simulink model "detumbling"  (R2020b)
settings: Solver=ode15s  StartTime=0  StopTime=10000  MaxStep=0.1  RelTol=1e-8  AbsTol=1e-8
values from neighbouring files (symbols this model uses):
  data = struct()    [config.m]    (also in config6U.m; configSlew.m; mainOffNominal.m = dataFix)
libraries: simulink_extras x1
settings Model: SimulationMode=accelerator  Creator=pacif  LastModifiedBy=pacif

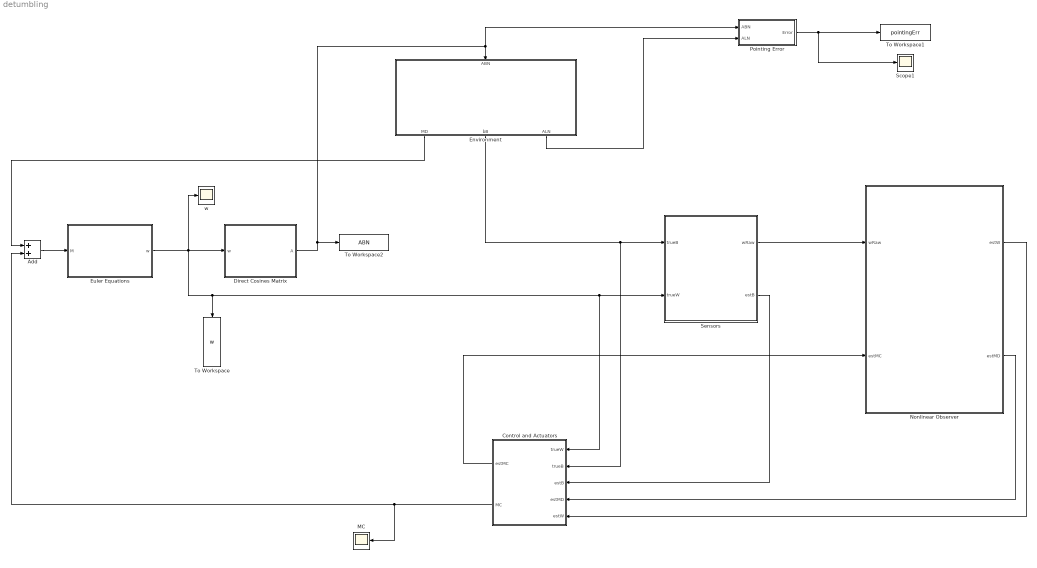
== system detumbling ==
  Add : Sum
  Control and Actuators : Subsystem
  Direct Cosines Matrix : Subsystem
  Environment : Subsystem
  Euler Equations : Subsystem
  MC : Scope
  Nonlinear Observer : Subsystem
  Pointing Error : Subsystem
  Scope1 : Scope
  Sensors : Subsystem
  To Workspace : ToWorkspace  VariableName=w  SaveFormat=Timeseries  SampleTime=-1
  To Workspace1 : ToWorkspace  VariableName=pointingErr  SaveFormat=Timeseries  SampleTime=-1
  To Workspace2 : ToWorkspace  VariableName=ABN  SaveFormat=Timeseries  SampleTime=-1
  w : Scope
  wires:
  Environment/2(bB) -> Sensors/1(trueB), Control and Actuators/2(trueB)
  Add/1 -> Euler Equations/1(M)
  Environment/1(MD) -> Add/1
  Control and Actuators/2(MC) -> MC/1, Add/2
  Sensors/2(estB) -> Control and Actuators/3(estB)
  Sensors/1(wRaw) -> Nonlinear Observer/1(wRaw)
  Control and Actuators/1(estMC) -> Nonlinear Observer/2(estMC)
  Nonlinear Observer/2(estMD) -> Control and Actuators/4(estMD)
  Euler Equations/1(w) -> w/1, Direct Cosines Matrix/1(w), To Workspace/1, Control and Actuators/1(trueW), Sensors/2(trueW)
  Nonlinear Observer/1(estW) -> Control and Actuators/5(estW)
  Pointing Error/1(Error) -> Scope1/1, To Workspace1/1
  Environment/3(ALN) -> Pointing Error/2(ALN)
  Direct Cosines Matrix/1(A) -> Pointing Error/1(ABN), Environment/1(ABN), To Workspace2/1

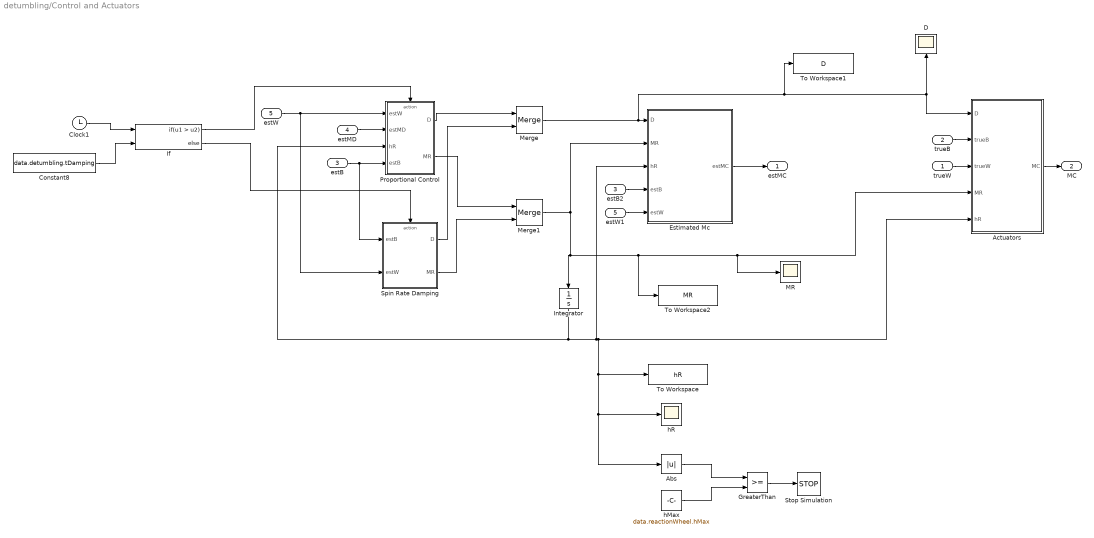
== system detumbling/Control and Actuators ==
  trueW : Inport
  trueB : Inport  Port=2
  estB : Inport  Port=3
  estMD : Inport  Port=4
  estW : Inport  Port=5
  Abs : Abs
  Actuators : Subsystem
  Clock1 : Clock
  Constant8 : Constant  Value=data.detumbling.tDamping
  D : Scope
  Estimated Mc : Subsystem
  GreaterThan : RelationalOperator  OutDataTypeStr=boolean  RndMeth=Simplest
  If : If  NumInputs=2  IfExpression=u1 > u2
  Integrator : Integrator  InitialCondition=data.reactionWheel.h0
  MR : Scope
  Merge : Merge
  Merge1 : Merge
  Proportional Control : Subsystem  TreatAsAtomicUnit=on
  Spin Rate Damping : Subsystem  TreatAsAtomicUnit=on
  Stop Simulation : Stop
  To Workspace : ToWorkspace  VariableName=hR  SaveFormat=Timeseries  SampleTime=-1
  To Workspace1 : ToWorkspace  VariableName=D  SaveFormat=Timeseries  SampleTime=-1
  To Workspace2 : ToWorkspace  VariableName=MR  SaveFormat=Timeseries  SampleTime=-1
  estB2 : InportShadow  Port=3
  estW1 : InportShadow  Port=5
  hMax : Constant  Value=data.reactionWheel.hMax
  hR : Scope
  estMC : Outport
  MC : Outport  Port=2
  wires:
  trueB/1 -> Actuators/2(trueB)
  Actuators/1(MC) -> MC/1
  trueW/1 -> Actuators/3(trueW)
  Merge/1 -> To Workspace1/1, Actuators/1(D), D/1, Estimated Mc/1(D)
  Estimated Mc/1(estMC) -> estMC/1
  Merge1/1 -> To Workspace2/1, Actuators/4(MR), MR/1, Integrator/1, Estimated Mc/2(MR)
  Spin Rate Damping/1(D) -> Merge/2
  Constant8/1 -> If/2
  If/2 -> Spin Rate Damping/Action
  Proportional Control/2(MR) -> Merge1/1
  estB/1 -> Spin Rate Damping/1(estB), Proportional Control/4(estB)
  estW/1 -> Proportional Control/1(estW), Spin Rate Damping/2(estW)
  Clock1/1 -> If/1
  If/1 -> Proportional Control/Action
  estMD/1 -> Proportional Control/2(estMD)
  Proportional Control/1(D) -> Merge/1
  Spin Rate Damping/2(MR) -> Merge1/2
  estB2/1 -> Estimated Mc/4(estB)
  estW1/1 -> Estimated Mc/5(estW)
  Abs/1 -> GreaterThan/1
  GreaterThan/1 -> Stop Simulation/1
  hMax/1 -> GreaterThan/2
  Integrator/1 -> Actuators/5(hR), To Workspace/1, Abs/1, hR/1, Estimated Mc/3(hR), Proportional Control/3(hR)

== system detumbling/Direct Cosines Matrix ==
  w : Inport
  Build 3x3 Matrix : Subsystem
  Constant1 : Constant  Value=0
  Demux1 : Demux  Outputs=3
  Gain{3,5..7} (4 alike) : Gain  Gain=-1
  Integrator : Integrator  InitialCondition=data.ic.dcm
  Orthonormalization : Subsystem
  Product : Product  Multiplication=Matrix(*)
  A : Outport
  wires:
  Demux1/1 -> Build 3x3 Matrix/6(A32), Gain7/1
  Gain5/1 -> Build 3x3 Matrix/4(A12)
  Demux1/3 -> Build 3x3 Matrix/2(A21), Gain5/1
  Product/1 -> Gain3/1
  Build 3x3 Matrix/1(A) -> Product/1  "[w]^"
  Gain6/1 -> Build 3x3 Matrix/3(A31)
  Demux1/2 -> Build 3x3 Matrix/7("A13 "), Gain6/1
  Gain7/1 -> Build 3x3 Matrix/8(A23)
  Orthonormalization/1(A) -> Product/2, A/1
  Gain3/1 -> Integrator/1  "dA/dt"
  w/1 -> Demux1/1
  Integrator/1 -> Orthonormalization/1(A0)  "A"
  Constant1/1 -> Build 3x3 Matrix/1(A11), Build 3x3 Matrix/9(A33), Build 3x3 Matrix/5(A22)

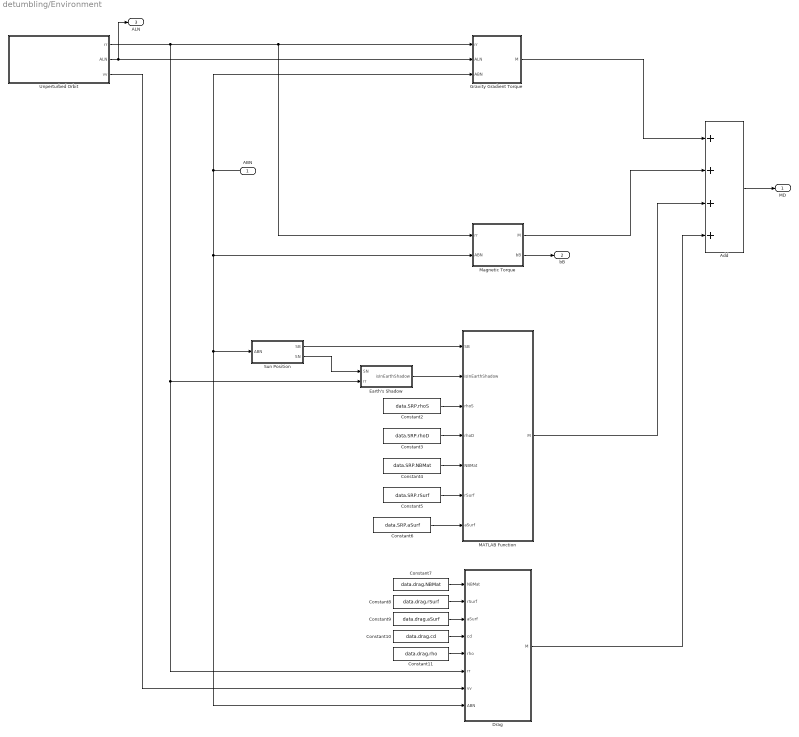
== system detumbling/Environment ==
  ABN : Inport
  Add : Sum  Inputs=++++
  Constant10 : Constant  Value=data.drag.cd
  Constant11 : Constant  Value=data.drag.rho
  Constant2 : Constant  Value=data.SRP.rhoS
  Constant3 : Constant  Value=data.SRP.rhoD
  Constant4 : Constant  Value=data.SRP.NBMat
  Constant5 : Constant  Value=data.SRP.rSurf
  Constant6 : Constant  Value=data.SRP.aSurf
  Constant7 : Constant  Value=data.drag.NBMat
  Constant8 : Constant  Value=data.drag.rSurf
  Constant9 : Constant  Value=data.drag.aSurf
  Drag : MATLAB Function  TreatAsAtomicUnit=on
  Earth's Shadow : Subsystem
  Gravity Gradient Torque : Subsystem
  MATLAB Function : MATLAB Function  TreatAsAtomicUnit=on
  Magnetic Torque : Subsystem
  "Sun Position " : Subsystem
  Unperturbed Orbit : Subsystem
  MD : Outport
  bB : Outport  Port=2
  ALN : Outport  Port=3
  wires:
  Earth's Shadow/1(isInEarthShadow) -> MATLAB Function/2(isInEarthShadow)
  "Sun Position "/1(SB) -> MATLAB Function/1(SB)
  Constant5/1 -> MATLAB Function/6(rSurf)
  Constant6/1 -> MATLAB Function/7(aSurf)
  Constant3/1 -> MATLAB Function/4(rhoD)
  Constant4/1 -> MATLAB Function/5(NBMat)
  Gravity Gradient Torque/1(M) -> Add/1
  Unperturbed Orbit/1(rr) -> Earth's Shadow/2(rr), Drag/6(rr), Magnetic Torque/1(rr), Gravity Gradient Torque/1(rr)
  MATLAB Function/1(M) -> Add/3
  Constant10/1 -> Drag/4(cd)
  Drag/1(M) -> Add/4
  ABN/1 -> Gravity Gradient Torque/3(ABN), Magnetic Torque/2(ABN), Drag/8(ABN), "Sun Position "/1(ABN)
  Constant7/1 -> Drag/1(NBMat)
  Constant8/1 -> Drag/2(rSurf)
  Constant9/1 -> Drag/3(aSurf)
  Add/1 -> MD/1
  Constant2/1 -> MATLAB Function/3(rhoS)
  Magnetic Torque/1(M) -> Add/2
  Unperturbed Orbit/2(ALN) -> Gravity Gradient Torque/2(ALN), ALN/1
  Constant11/1 -> Drag/5(rho)
  Unperturbed Orbit/3(vv) -> Drag/7(vv)
  Magnetic Torque/2(bB) -> bB/1
  "Sun Position "/2(SN) -> Earth's Shadow/1(SN)

== system detumbling/Euler Equations ==
  M : Inport
  Add : Sum
  Cross Product : Subsystem
  Gain : Gain  Gain=data.sc.invI  Multiplication=Matrix(K*u) (u vector)
  Gain2 : Gain  Gain=data.sc.inertiaMatrix  Multiplication=Matrix(K*u) (u vector)
  Integrator : Integrator  InitialCondition=data.ic.w
  w : Outport
  wires:
  Gain2/1 -> Cross Product/1(a)  "I*w"
  Cross Product/1(c) -> Add/2  "I*w x w = -w x I*w"
  M/1 -> Add/1
  Integrator/1 -> Cross Product/2(b), Gain2/1, w/1  "w"
  Gain/1 -> Integrator/1  "dw"
  Add/1 -> Gain/1

== system detumbling/Nonlinear Observer ==
  wRaw : Inport
  estMC : Inport  Port=2
  Observer : Subsystem
  estW : Outport
  estMD : Outport  Port=2
  wires:
  wRaw/1 -> Observer/1(wRaw)
  estMC/1 -> Observer/2(estMC)
  Observer/1(estW) -> estW/1
  Observer/2(estMD) -> estMD/1

== system detumbling/Pointing Error ==
  ABN : Inport
  ALN : Inport  Port=2
  Acos : Trigonometry  Operator=acos
  Product : Product  Multiplication=Matrix(*)
  Radians to Degrees : simulink_extras/Transformations/Radians to Degrees
  Selector : Selector  NumberOfDimensions=2  InputPortWidth=3  IndexOptions=Index vector (dialog),Index vector (dialog)  Indices=1,1  OutputSizes=1,1
  Transpose : Math  Operator=transpose  SaturateOnIntegerOverflow=on
  Error : Outport
  wires:
  Radians to Degrees/1 -> Error/1
  ABN/1 -> Product/1
  ALN/1 -> Transpose/1
  Transpose/1 -> Product/2
  Product/1 -> Selector/1
  Selector/1 -> Acos/1
  Acos/1 -> Radians to Degrees/1

== system detumbling/Sensors ==
  trueB : Inport
  trueW : Inport  Port=2
  Add3 : Sum  Inputs=+-
  Gyro Error : Scope
  Gyroscope : Subsystem
  Magnetometer : Subsystem
  wRaw : Outport
  estB : Outport  Port=2
  wires:
  Gyroscope/1(wRaw) -> wRaw/1, Add3/2
  trueW/1 -> Add3/1, Gyroscope/1(trueW)
  Add3/1 -> Gyro Error/1
  Magnetometer/1(estB) -> estB/1
  trueB/1 -> Magnetometer/1(B)

== system detumbling/Control and Actuators/Actuators ==
  D : Inport
  trueB : Inport  Port=2
  trueW : Inport  Port=3
  MR : Inport  Port=4
  hR : Inport  Port=5
  Add : Sum
  Add1 : Sum
  Cross Product : Subsystem
  Cross Product1 : Subsystem
  Gain : Gain  Gain=-1
  Product : Product
  Product1 : Product
  Reaction Wheel Axis : Constant  Value=data.reactionWheel.axis
  MC : Outport
  wires:
  D/1 -> Cross Product/1(a)
  trueB/1 -> Cross Product/2(b)
  Add/1 -> MC/1
  Cross Product/1(c) -> Add/1
  Gain/1 -> Add/2
  Add1/1 -> Gain/1
  Cross Product1/1(c) -> Add1/1
  trueW/1 -> Cross Product1/1(a)
  Product/1 -> Cross Product1/2(b)
  MR/1 -> Product1/2
  hR/1 -> Product/1
  Reaction Wheel Axis/1 -> Product1/1, Product/2
  Product1/1 -> Add1/2

== system detumbling/Control and Actuators/Estimated Mc ==
  D : Inport
  MR : Inport  Port=2
  hR : Inport  Port=3
  estB : Inport  Port=4
  estW : Inport  Port=5
  Add : Sum  Inputs=+--
  Cross Product : Subsystem
  Cross Product1 : Subsystem
  Product : Product
  Product1 : Product
  RW Axis : Constant  Value=data.reactionWheel.axis
  RW Axis1 : Constant  Value=data.reactionWheel.axis
  estMC : Outport
  wires:
  D/1 -> Cross Product/1(a)
  estB/1 -> Cross Product/2(b)
  Add/1 -> estMC/1
  Cross Product/1(c) -> Add/1
  RW Axis/1 -> Product/1
  MR/1 -> Product/2
  Product/1 -> Add/2
  Cross Product1/1(c) -> Add/3
  estW/1 -> Cross Product1/1(a)
  hR/1 -> Product1/2
  RW Axis1/1 -> Product1/1
  Product1/1 -> Cross Product1/2(b)

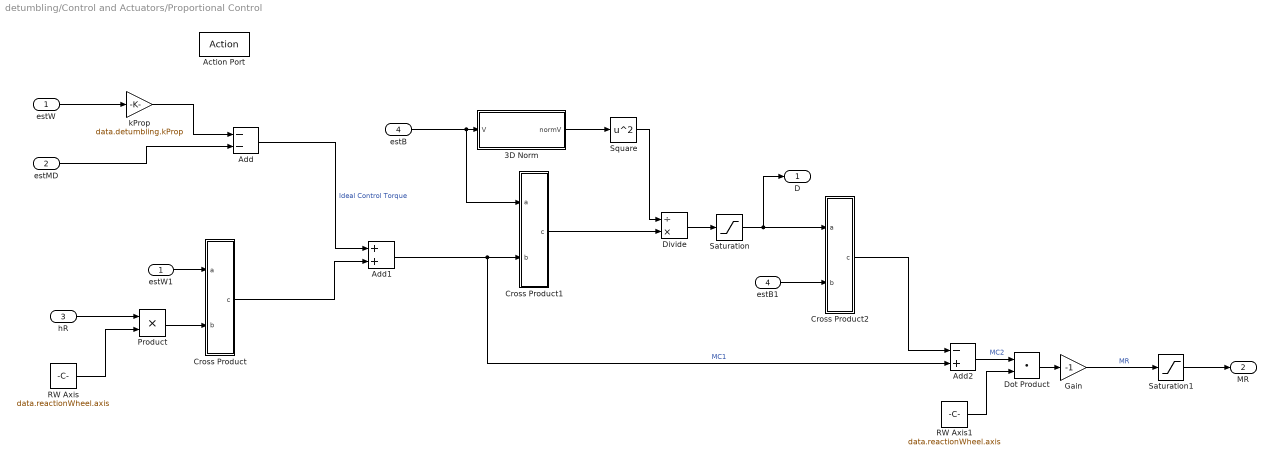
== system detumbling/Control and Actuators/Proportional Control ==
  estW : Inport
  estMD : Inport  Port=2
  hR : Inport  Port=3
  estB : Inport  Port=4
  Action Port : ActionPort  ActionPortLabel=if(u1 > u2)
  3D Norm : Subsystem
  Add : Sum  Inputs=--
  Add1 : Sum
  Add2 : Sum  Inputs=-+
  Cross Product : Subsystem
  Cross Product1 : Subsystem
  Cross Product2 : Subsystem
  Divide : Product  Inputs=/*
  Dot Product : DotProduct  InputSameDT=on  OutDataTypeStr=Inherit: Inherit via internal rule
  Gain : Gain  Gain=-1
  Product : Product
  RW Axis : Constant  Value=data.reactionWheel.axis
  RW Axis1 : Constant  Value=data.reactionWheel.axis
  Saturation : Saturate  UpperLimit=data.magnetorquer.DMax  LowerLimit=-data.magnetorquer.DMax  LinearizeAsGain=off
  Saturation1 : Saturate  UpperLimit=data.reactionWheel.MMax  LowerLimit=-data.reactionWheel.MMax
  Square : Math  Operator=square  SaturateOnIntegerOverflow=on
  estB1 : InportShadow  Port=4
  estW1 : InportShadow
  kProp : Gain  Gain=data.detumbling.kProp
  D : Outport
  MR : Outport  Port=2
  wires:
  Saturation/1 -> Cross Product2/1(a), D/1
  Divide/1 -> Saturation/1
  estW/1 -> kProp/1
  kProp/1 -> Add/1
  estMD/1 -> Add/2
  Add/1 -> Add1/1  "Ideal Control Torque"
  estW1/1 -> Cross Product/1(a)
  Product/1 -> Cross Product/2(b)
  hR/1 -> Product/1
  RW Axis/1 -> Product/2
  Cross Product/1(c) -> Add1/2
  estB/1 -> Cross Product1/1(a), 3D Norm/1(V)
  3D Norm/1(normV) -> Square/1
  Add1/1 -> Cross Product1/2(b), Add2/2  "MC1"
  Cross Product1/1(c) -> Divide/2
  Square/1 -> Divide/1
  estB1/1 -> Cross Product2/2(b)
  Cross Product2/1(c) -> Add2/1
  Add2/1 -> Dot Product/1  "MC2"
  Dot Product/1 -> Gain/1
  RW Axis1/1 -> Dot Product/2
  Gain/1 -> Saturation1/1  "MR"
  Saturation1/1 -> MR/1

== system detumbling/Control and Actuators/Spin Rate Damping ==
  estB : Inport
  estW : Inport  Port=2
  Action Port : ActionPort  ActionPortLabel=else
  Constant : Constant  Value=0
  Cross Product1 : Subsystem
  Saturation : Saturate  UpperLimit=data.magnetorquer.DMax  LowerLimit=-data.magnetorquer.DMax  LinearizeAsGain=off
  k : Gain  Gain=data.detumbling.kDamping
  D : Outport
  MR : Outport  Port=2
  wires:
  estW/1 -> Cross Product1/1(a)
  estB/1 -> Cross Product1/2(b)
  Cross Product1/1(c) -> k/1
  k/1 -> Saturation/1
  Constant/1 -> MR/1
  Saturation/1 -> D/1

== system detumbling/Direct Cosines Matrix/Build 3x3 Matrix ==
  A11 : Inport
  A21 : Inport  Port=2
  A31 : Inport  Port=3
  A12 : Inport  Port=4
  A22 : Inport  Port=5
  A32 : Inport  Port=6
  "A13 " : Inport  Port=7
  A23 : Inport  Port=8
  A33 : Inport  Port=9
  Mux : Mux  Inputs=3
  Mux1 : Mux  Inputs=3
  Mux2 : Mux  Inputs=3
  Vector Concatenate : Concatenate  NumInputs=3  Mode=Multidimensional array  ConcatenateDimension=2
  A : Outport
  wires:
  A21/1 -> Mux/2
  A23/1 -> Mux2/2
  "A13 "/1 -> Mux2/1
  A11/1 -> Mux/1
  Vector Concatenate/1 -> A/1
  A31/1 -> Mux/3
  A12/1 -> Mux1/1
  A22/1 -> Mux1/2
  Mux2/1 -> Vector Concatenate/3
  Mux1/1 -> Vector Concatenate/2
  Mux/1 -> Vector Concatenate/1
  A33/1 -> Mux2/3
  A32/1 -> Mux1/3

== system detumbling/Direct Cosines Matrix/Orthonormalization ==
  A0 : Inport
  Add : Sum  Inputs=+-
  Gain : Gain  Gain=1.5
  Gain1 : Gain  Gain=0.5
  Product : Product  Inputs=3  Multiplication=Matrix(*)
  Transpose : Math  Operator=transpose  SaturateOnIntegerOverflow=on
  A : Outport
  wires:
  Add/1 -> A/1
  A0/1 -> Product/3, Transpose/1, Product/1, Gain/1
  Gain1/1 -> Add/2
  Gain/1 -> Add/1
  Transpose/1 -> Product/2
  Product/1 -> Gain1/1

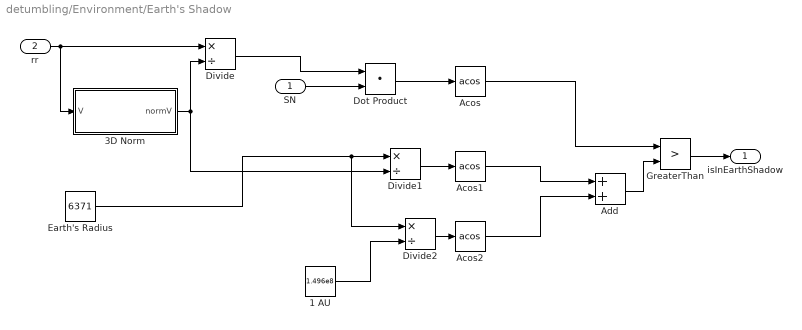
== system detumbling/Environment/Earth's Shadow ==
  SN : Inport
  rr : Inport  Port=2
  1 AU : Constant  Value=1.496e8
  3D Norm : Subsystem
  Acos : Trigonometry  Operator=acos
  Acos1 : Trigonometry  Operator=acos
  Acos2 : Trigonometry  Operator=acos
  Add : Sum
  Divide : Product  Inputs=*/
  Divide1 : Product  Inputs=*/
  Divide2 : Product  Inputs=*/
  Dot Product : DotProduct  InputSameDT=on  OutDataTypeStr=Inherit: Inherit via internal rule
  Earth's Radius : Constant  Value=6371
  GreaterThan : RelationalOperator  Operator=>  OutDataTypeStr=boolean  RndMeth=Simplest
  isInEarthShadow : Outport
  wires:
  SN/1 -> Dot Product/2
  GreaterThan/1 -> isInEarthShadow/1
  Add/1 -> GreaterThan/2
  Acos/1 -> GreaterThan/1
  Acos2/1 -> Add/2
  Acos1/1 -> Add/1
  rr/1 -> 3D Norm/1(V), Divide/1
  3D Norm/1(normV) -> Divide1/2, Divide/2
  Divide/1 -> Dot Product/1
  Dot Product/1 -> Acos/1
  Earth's Radius/1 -> Divide1/1, Divide2/1
  Divide1/1 -> Acos1/1
  Divide2/1 -> Acos2/1
  1 AU/1 -> Divide2/2

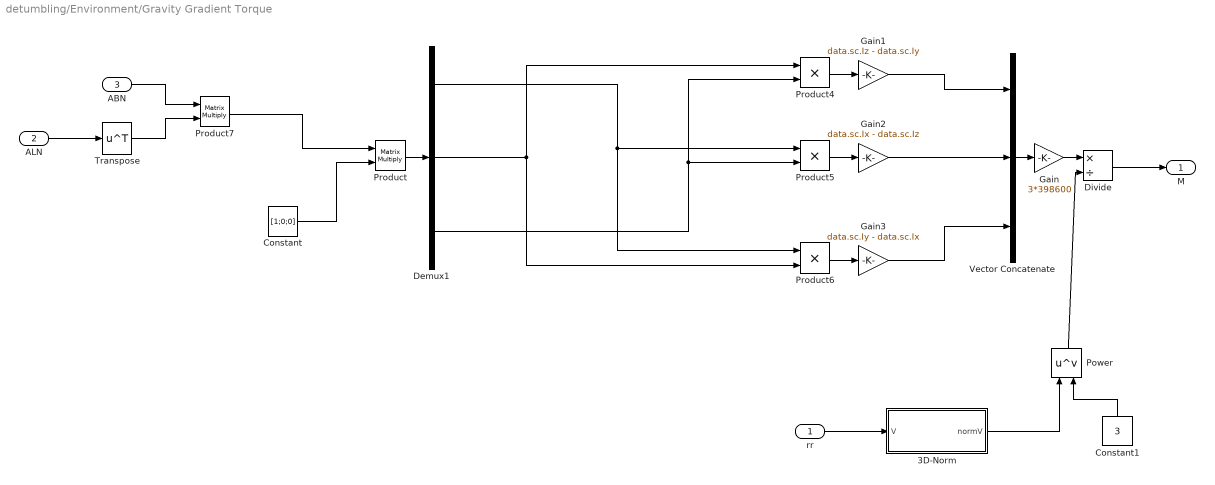
== system detumbling/Environment/Gravity Gradient Torque ==
  rr : Inport
  ALN : Inport  Port=2
  ABN : Inport  Port=3
  3D-Norm : Subsystem
  Constant : Constant  Value=[1;0;0]  VectorParams1D=off
  Constant1 : Constant  Value=3
  Demux1 : Demux  Outputs=3
  Divide : Product  Inputs=*/
  Gain : Gain  Gain=3*398600
  Gain1 : Gain  Gain=data.sc.Iz - data.sc.Iy
  Gain2 : Gain  Gain=data.sc.Ix - data.sc.Iz
  Gain3 : Gain  Gain=data.sc.Iy - data.sc.Ix
  Power : Math  Operator=pow  SaturateOnIntegerOverflow=on
  Product : Product  Multiplication=Matrix(*)
  Product4 : Product
  Product5 : Product
  Product6 : Product
  Product7 : Product  Multiplication=Matrix(*)
  Transpose : Math  Operator=transpose  SaturateOnIntegerOverflow=on
  Vector Concatenate : Concatenate  NumInputs=3
  M : Outport
  wires:
  Constant/1 -> Product/2
  Gain3/1 -> Vector Concatenate/3
  Gain1/1 -> Vector Concatenate/1
  Gain2/1 -> Vector Concatenate/2
  Vector Concatenate/1 -> Gain/1
  Constant1/1 -> Power/2
  Power/1 -> Divide/2
  Gain/1 -> Divide/1
  Product/1 -> Demux1/1
  Product4/1 -> Gain1/1
  Product5/1 -> Gain2/1
  Product6/1 -> Gain3/1
  Demux1/1 -> Product6/1, Product5/1
  Demux1/2 -> Product6/2, Product4/1
  Demux1/3 -> Product5/2, Product4/2
  Divide/1 -> M/1
  rr/1 -> 3D-Norm/1(V)
  3D-Norm/1(normV) -> Power/1
  ALN/1 -> Transpose/1
  Product7/1 -> Product/1
  ABN/1 -> Product7/1
  Transpose/1 -> Product7/2

== system detumbling/Environment/Magnetic Torque ==
  rr : Inport
  ABN : Inport  Port=2
  Cross Product : Subsystem
  Product : Product  Multiplication=Matrix(*)
  Subsystem : Subsystem
  m : Constant  Value=data.magneticTorque.m
  M : Outport
  bB : Outport  Port=2
  wires:
  rr/1 -> Subsystem/1(rr)
  ABN/1 -> Product/1
  Subsystem/1(bN) -> Product/2
  m/1 -> Cross Product/1(a)
  Product/1 -> Cross Product/2(b), bB/1
  Cross Product/1(c) -> M/1

== system detumbling/Environment/Sun Position  ==
  ABN : Inport
  Clock : Clock
  Cos : Trigonometry  Operator=cos
  Gain1 : Gain  Gain=2*pi/365/24/3600
  Gain2 : Gain  Gain=cos(23.45*pi/180)
  Gain3 : Gain  Gain=sin(23.45*pi/180)
  Mux : Mux  Inputs=3
  Product : Product  Multiplication=Matrix(*)
  Sin : Trigonometry
  Sin1 : Trigonometry
  SB : Outport
  SN : Outport  Port=2
  wires:
  Clock/1 -> Gain1/1
  Mux/1 -> SN/1, Product/2  "SN"
  Gain2/1 -> Mux/2
  Gain3/1 -> Mux/3
  Cos/1 -> Mux/1
  Sin1/1 -> Gain3/1
  Sin/1 -> Gain2/1
  Gain1/1 -> Sin/1, Sin1/1, Cos/1
  ABN/1 -> Product/1
  Product/1 -> SB/1

== system detumbling/Environment/Unperturbed Orbit ==
  Integrator : Integrator  InitialCondition=data.ic.th
  Subsystem : Subsystem
  Subsystem1 : Subsystem
  Subsystem2 : Subsystem
  Subsystem3 : Subsystem
  To Workspace : ToWorkspace  VariableName=theta  SaveFormat=Timeseries  SampleTime=-1
  rr : Outport
  ALN : Outport  Port=2
  vv : Outport  Port=3
  wires:
  Subsystem2/1(rr) -> rr/1
  Subsystem/1(theta_dot) -> Integrator/1
  Subsystem1/1(ALN) -> ALN/1
  Subsystem3/1(vv) -> vv/1
  Integrator/1 -> Subsystem2/1(theta), Subsystem1/1(theta), Subsystem3/1(theta), To Workspace/1, Subsystem/1(theta)

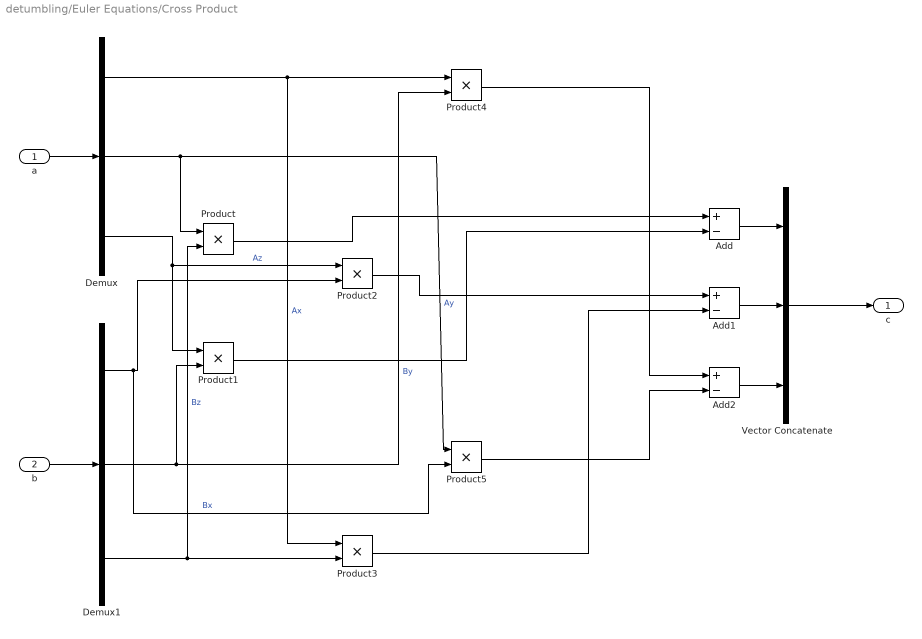
== system detumbling/Euler Equations/Cross Product ==
  a : Inport
  b : Inport  Port=2
  Add : Sum  Inputs=+-
  Add1 : Sum  Inputs=+-
  Add2 : Sum  Inputs=+-
  Demux : Demux  Outputs=3
  Demux1 : Demux  Outputs=3
  Product{,1..5} (6 alike) : Product
  Vector Concatenate : Concatenate  NumInputs=3
  c : Outport
  wires:
  Demux1/1 -> Product2/2, Product5/2  "Bx"
  Product2/1 -> Add1/1
  Vector Concatenate/1 -> c/1
  Add/1 -> Vector Concatenate/1
  Product3/1 -> Add1/2
  Product1/1 -> Add/2
  Product4/1 -> Add2/1
  Product/1 -> Add/1
  Demux/1 -> Product3/1, Product4/1  "Ax"
  Product5/1 -> Add2/2
  Demux/3 -> Product2/1, Product1/1  "Az"
  b/1 -> Demux1/1
  a/1 -> Demux/1
  Add2/1 -> Vector Concatenate/3
  Demux/2 -> Product5/1, Product/1  "Ay"
  Demux1/3 -> Product/2, Product3/2  "Bz"
  Demux1/2 -> Product4/2, Product1/2  "By"
  Add1/1 -> Vector Concatenate/2

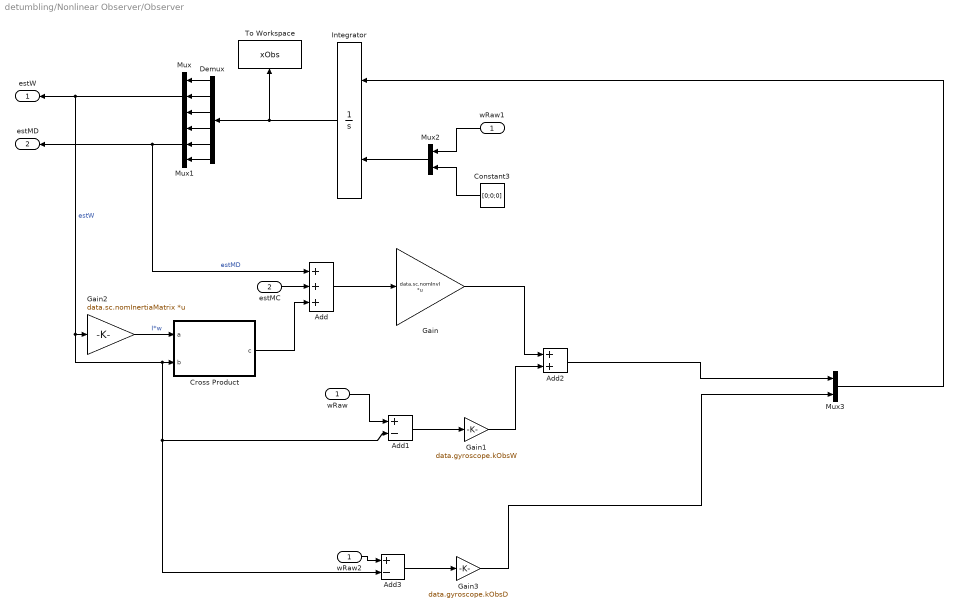
== system detumbling/Nonlinear Observer/Observer ==
  wRaw : Inport
  estMC : Inport  Port=2
  Add : Sum  Inputs=+++
  Add1 : Sum  Inputs=+-
  Add2 : Sum
  Add3 : Sum  Inputs=+-
  Constant3 : Constant  Value=[0;0;0]
  Cross Product : Subsystem
  Demux : Demux  Outputs=6
  Gain : Gain  Gain=data.sc.nomInvI  Multiplication=Matrix(K*u) (u vector)
  Gain1 : Gain  Gain=data.gyroscope.kObsW
  Gain2 : Gain  Gain=data.sc.nomInertiaMatrix  Multiplication=Matrix(K*u) (u vector)
  Gain3 : Gain  Gain=data.gyroscope.kObsD
  Integrator : Integrator  InitialConditionSource=external  InitialCondition=data.gyroscope.xObs0
  Mux : Mux  Inputs=3
  Mux1 : Mux  Inputs=3
  Mux2 : Mux  Inputs=2
  Mux3 : Mux  Inputs=2
  To Workspace : ToWorkspace  VariableName=xObs  SaveFormat=Timeseries  SampleTime=-1
  wRaw1 : InportShadow
  wRaw2 : InportShadow
  estW : Outport
  estMD : Outport  Port=2
  wires:
  Mux3/1 -> Integrator/1
  Integrator/1 -> Demux/1, To Workspace/1
  estMC/1 -> Add/2
  Demux/1 -> Mux/1
  Demux/2 -> Mux/2
  Demux/3 -> Mux/3
  Demux/5 -> Mux1/2
  Demux/4 -> Mux1/1
  Demux/6 -> Mux1/3
  Mux1/1 -> Add/1, estMD/1  "estMD"
  Mux2/1 -> Integrator/2
  wRaw1/1 -> Mux2/1
  Constant3/1 -> Mux2/2
  Cross Product/1(c) -> Add/3
  Add/1 -> Gain/1
  Gain2/1 -> Cross Product/1(a)  "I*w"
  Gain/1 -> Add2/1
  wRaw/1 -> Add1/1
  Add1/1 -> Gain1/1
  Gain1/1 -> Add2/2
  Add2/1 -> Mux3/1
  Add3/1 -> Gain3/1
  Mux/1 -> Add3/2, Add1/2, Cross Product/2(b), Gain2/1, estW/1  "estW"
  Gain3/1 -> Mux3/2
  wRaw2/1 -> Add3/1

== system detumbling/Sensors/Gyroscope ==
  trueW : Inport
  Add : Sum
  Add1 : Sum
  Integrator : Integrator  InitialCondition=data.gyroscope.b0
  Random Number : RandomNumber  Variance=data.gyroscope.sigmaN^2*[1;1;1]  Seed=[2323; 3445;34]  SampleTime=data.gyroscope.sampleTime
  Random Number1 : RandomNumber  Variance=data.gyroscope.sigmaB^2*[1;1;1]  Seed=[34432; 345456;1087]  SampleTime=data.gyroscope.sampleTime
  To Workspace : ToWorkspace  VariableName=bGyro  SaveFormat=Timeseries  SampleTime=-1
  Zero-Order Hold : ZeroOrderHold  SampleTime=data.gyroscope.sampleTime
  wRaw : Outport
  wires:
  Zero-Order Hold/1 -> wRaw/1
  Add/1 -> Zero-Order Hold/1
  Random Number/1 -> Add1/1
  Add1/1 -> Add/2
  trueW/1 -> Add/1
  Integrator/1 -> To Workspace/1, Add1/2
  Random Number1/1 -> Integrator/1

== system detumbling/Sensors/Magnetometer ==
  B : Inport
  Add : Sum
  Multiply : Gain  Gain=data.magnetometer.nonOrthogonality  Multiplication=Matrix(K*u) (u vector)
  Random Number1 : RandomNumber  Variance=(data.magnetometer.sigma)^2*[1;1;1]  Seed=randi(1e5,3,1)  SampleTime=data.magnetometer.sampleTime
  Zero-Order Hold : ZeroOrderHold  SampleTime=data.magnetometer.sampleTime
  estB : Outport
  wires:
  Random Number1/1 -> Add/2
  Add/1 -> Zero-Order Hold/1
  B/1 -> Add/1
  Zero-Order Hold/1 -> Multiply/1
  Multiply/1 -> estB/1

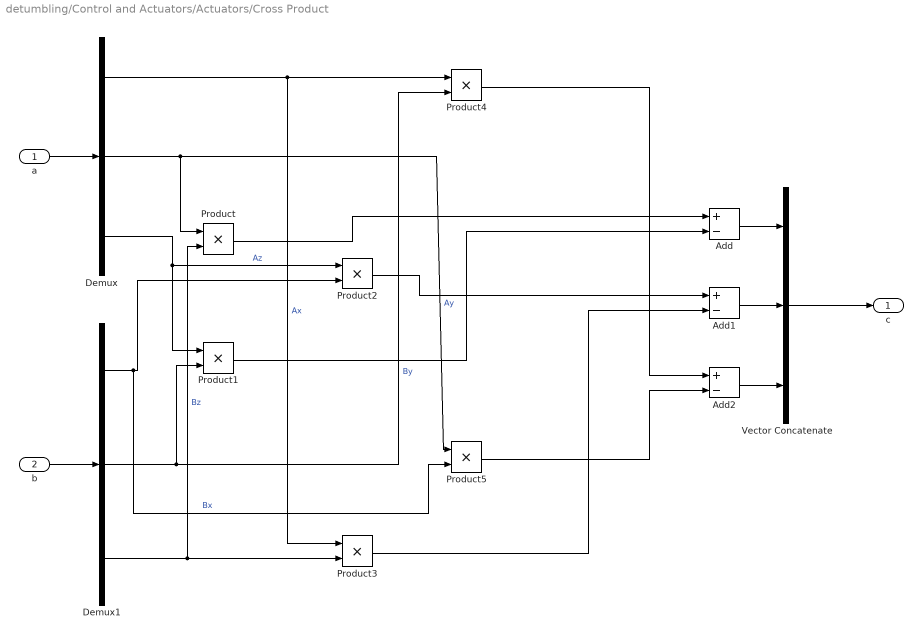
== system detumbling/Control and Actuators/Actuators/Cross Product ==
  a : Inport
  b : Inport  Port=2
  Add : Sum  Inputs=+-
  Add1 : Sum  Inputs=+-
  Add2 : Sum  Inputs=+-
  Demux : Demux  Outputs=3
  Demux1 : Demux  Outputs=3
  Product{,1..5} (6 alike) : Product
  Vector Concatenate : Concatenate  NumInputs=3
  c : Outport
  wires:
  Demux1/1 -> Product2/2, Product5/2  "Bx"
  Product2/1 -> Add1/1
  Vector Concatenate/1 -> c/1
  Add/1 -> Vector Concatenate/1
  Product3/1 -> Add1/2
  Product1/1 -> Add/2
  Product4/1 -> Add2/1
  Product/1 -> Add/1
  Demux/1 -> Product3/1, Product4/1  "Ax"
  Product5/1 -> Add2/2
  Demux/3 -> Product2/1, Product1/1  "Az"
  b/1 -> Demux1/1
  a/1 -> Demux/1
  Add2/1 -> Vector Concatenate/3
  Demux/2 -> Product5/1, Product/1  "Ay"
  Demux1/3 -> Product/2, Product3/2  "Bz"
  Demux1/2 -> Product4/2, Product1/2  "By"
  Add1/1 -> Vector Concatenate/2

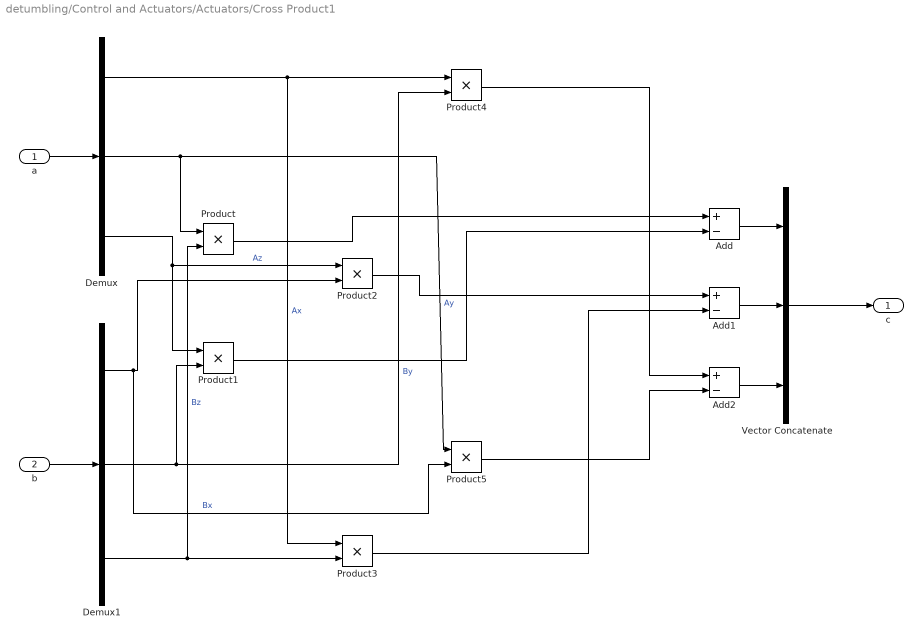
== system detumbling/Control and Actuators/Actuators/Cross Product1 ==
  a : Inport
  b : Inport  Port=2
  Add : Sum  Inputs=+-
  Add1 : Sum  Inputs=+-
  Add2 : Sum  Inputs=+-
  Demux : Demux  Outputs=3
  Demux1 : Demux  Outputs=3
  Product{,1..5} (6 alike) : Product
  Vector Concatenate : Concatenate  NumInputs=3
  c : Outport
  wires:
  Demux1/1 -> Product2/2, Product5/2  "Bx"
  Product2/1 -> Add1/1
  Vector Concatenate/1 -> c/1
  Add/1 -> Vector Concatenate/1
  Product3/1 -> Add1/2
  Product1/1 -> Add/2
  Product4/1 -> Add2/1
  Product/1 -> Add/1
  Demux/1 -> Product3/1, Product4/1  "Ax"
  Product5/1 -> Add2/2
  Demux/3 -> Product2/1, Product1/1  "Az"
  b/1 -> Demux1/1
  a/1 -> Demux/1
  Add2/1 -> Vector Concatenate/3
  Demux/2 -> Product5/1, Product/1  "Ay"
  Demux1/3 -> Product/2, Product3/2  "Bz"
  Demux1/2 -> Product4/2, Product1/2  "By"
  Add1/1 -> Vector Concatenate/2

== system detumbling/Control and Actuators/Estimated Mc/Cross Product ==
  a : Inport
  b : Inport  Port=2
  Add : Sum  Inputs=+-
  Add1 : Sum  Inputs=+-
  Add2 : Sum  Inputs=+-
  Demux : Demux  Outputs=3
  Demux1 : Demux  Outputs=3
  Product{,1..5} (6 alike) : Product
  Vector Concatenate : Concatenate  NumInputs=3
  c : Outport
  wires:
  Demux1/1 -> Product2/2, Product5/2  "Bx"
  Product2/1 -> Add1/1
  Vector Concatenate/1 -> c/1
  Add/1 -> Vector Concatenate/1
  Product3/1 -> Add1/2
  Product1/1 -> Add/2
  Product4/1 -> Add2/1
  Product/1 -> Add/1
  Demux/1 -> Product3/1, Product4/1  "Ax"
  Product5/1 -> Add2/2
  Demux/3 -> Product2/1, Product1/1  "Az"
  b/1 -> Demux1/1
  a/1 -> Demux/1
  Add2/1 -> Vector Concatenate/3
  Demux/2 -> Product5/1, Product/1  "Ay"
  Demux1/3 -> Product/2, Product3/2  "Bz"
  Demux1/2 -> Product4/2, Product1/2  "By"
  Add1/1 -> Vector Concatenate/2

== system detumbling/Control and Actuators/Estimated Mc/Cross Product1 ==
  a : Inport
  b : Inport  Port=2
  Add : Sum  Inputs=+-
  Add1 : Sum  Inputs=+-
  Add2 : Sum  Inputs=+-
  Demux : Demux  Outputs=3
  Demux1 : Demux  Outputs=3
  Product{,1..5} (6 alike) : Product
  Vector Concatenate : Concatenate  NumInputs=3
  c : Outport
  wires:
  Demux1/1 -> Product2/2, Product5/2  "Bx"
  Product2/1 -> Add1/1
  Vector Concatenate/1 -> c/1
  Add/1 -> Vector Concatenate/1
  Product3/1 -> Add1/2
  Product1/1 -> Add/2
  Product4/1 -> Add2/1
  Product/1 -> Add/1
  Demux/1 -> Product3/1, Product4/1  "Ax"
  Product5/1 -> Add2/2
  Demux/3 -> Product2/1, Product1/1  "Az"
  b/1 -> Demux1/1
  a/1 -> Demux/1
  Add2/1 -> Vector Concatenate/3
  Demux/2 -> Product5/1, Product/1  "Ay"
  Demux1/3 -> Product/2, Product3/2  "Bz"
  Demux1/2 -> Product4/2, Product1/2  "By"
  Add1/1 -> Vector Concatenate/2

== system detumbling/Control and Actuators/Proportional Control/3D Norm ==
  V : Inport
  Add : Sum  Inputs=+++
  Demux : Demux  Outputs=3
  Square : Math  Operator=square  SaturateOnIntegerOverflow=on
  Square Root : Sqrt  SaturateOnIntegerOverflow=on
  Square1 : Math  Operator=square  SaturateOnIntegerOverflow=on
  Square2 : Math  Operator=square  SaturateOnIntegerOverflow=on
  normV : Outport
  wires:
  Square Root/1 -> normV/1
  V/1 -> Demux/1
  Demux/3 -> Square2/1
  Square/1 -> Add/1
  Demux/1 -> Square/1
  Demux/2 -> Square1/1
  Square2/1 -> Add/3
  Square1/1 -> Add/2
  Add/1 -> Square Root/1

== system detumbling/Control and Actuators/Proportional Control/Cross Product ==
  a : Inport
  b : Inport  Port=2
  Add : Sum  Inputs=+-
  Add1 : Sum  Inputs=+-
  Add2 : Sum  Inputs=+-
  Demux : Demux  Outputs=3
  Demux1 : Demux  Outputs=3
  Product{,1..5} (6 alike) : Product
  Vector Concatenate : Concatenate  NumInputs=3
  c : Outport
  wires:
  Demux1/1 -> Product2/2, Product5/2  "Bx"
  Product2/1 -> Add1/1
  Vector Concatenate/1 -> c/1
  Add/1 -> Vector Concatenate/1
  Product3/1 -> Add1/2
  Product1/1 -> Add/2
  Product4/1 -> Add2/1
  Product/1 -> Add/1
  Demux/1 -> Product3/1, Product4/1  "Ax"
  Product5/1 -> Add2/2
  Demux/3 -> Product2/1, Product1/1  "Az"
  b/1 -> Demux1/1
  a/1 -> Demux/1
  Add2/1 -> Vector Concatenate/3
  Demux/2 -> Product5/1, Product/1  "Ay"
  Demux1/3 -> Product/2, Product3/2  "Bz"
  Demux1/2 -> Product4/2, Product1/2  "By"
  Add1/1 -> Vector Concatenate/2

== system detumbling/Control and Actuators/Proportional Control/Cross Product1 ==
  a : Inport
  b : Inport  Port=2
  Add : Sum  Inputs=+-
  Add1 : Sum  Inputs=+-
  Add2 : Sum  Inputs=+-
  Demux : Demux  Outputs=3
  Demux1 : Demux  Outputs=3
  Product{,1..5} (6 alike) : Product
  Vector Concatenate : Concatenate  NumInputs=3
  c : Outport
  wires:
  Demux1/1 -> Product2/2, Product5/2  "Bx"
  Product2/1 -> Add1/1
  Vector Concatenate/1 -> c/1
  Add/1 -> Vector Concatenate/1
  Product3/1 -> Add1/2
  Product1/1 -> Add/2
  Product4/1 -> Add2/1
  Product/1 -> Add/1
  Demux/1 -> Product3/1, Product4/1  "Ax"
  Product5/1 -> Add2/2
  Demux/3 -> Product2/1, Product1/1  "Az"
  b/1 -> Demux1/1
  a/1 -> Demux/1
  Add2/1 -> Vector Concatenate/3
  Demux/2 -> Product5/1, Product/1  "Ay"
  Demux1/3 -> Product/2, Product3/2  "Bz"
  Demux1/2 -> Product4/2, Product1/2  "By"
  Add1/1 -> Vector Concatenate/2

== system detumbling/Control and Actuators/Proportional Control/Cross Product2 ==
  a : Inport
  b : Inport  Port=2
  Add : Sum  Inputs=+-
  Add1 : Sum  Inputs=+-
  Add2 : Sum  Inputs=+-
  Demux : Demux  Outputs=3
  Demux1 : Demux  Outputs=3
  Product{,1..5} (6 alike) : Product
  Vector Concatenate : Concatenate  NumInputs=3
  c : Outport
  wires:
  Demux1/1 -> Product2/2, Product5/2  "Bx"
  Product2/1 -> Add1/1
  Vector Concatenate/1 -> c/1
  Add/1 -> Vector Concatenate/1
  Product3/1 -> Add1/2
  Product1/1 -> Add/2
  Product4/1 -> Add2/1
  Product/1 -> Add/1
  Demux/1 -> Product3/1, Product4/1  "Ax"
  Product5/1 -> Add2/2
  Demux/3 -> Product2/1, Product1/1  "Az"
  b/1 -> Demux1/1
  a/1 -> Demux/1
  Add2/1 -> Vector Concatenate/3
  Demux/2 -> Product5/1, Product/1  "Ay"
  Demux1/3 -> Product/2, Product3/2  "Bz"
  Demux1/2 -> Product4/2, Product1/2  "By"
  Add1/1 -> Vector Concatenate/2

== system detumbling/Control and Actuators/Spin Rate Damping/Cross Product1 ==
  a : Inport
  b : Inport  Port=2
  Add : Sum  Inputs=+-
  Add1 : Sum  Inputs=+-
  Add2 : Sum  Inputs=+-
  Demux : Demux  Outputs=3
  Demux1 : Demux  Outputs=3
  Product{,1..5} (6 alike) : Product
  Vector Concatenate : Concatenate  NumInputs=3
  c : Outport
  wires:
  Demux1/1 -> Product2/2, Product5/2  "Bx"
  Product2/1 -> Add1/1
  Vector Concatenate/1 -> c/1
  Add/1 -> Vector Concatenate/1
  Product3/1 -> Add1/2
  Product1/1 -> Add/2
  Product4/1 -> Add2/1
  Product/1 -> Add/1
  Demux/1 -> Product3/1, Product4/1  "Ax"
  Product5/1 -> Add2/2
  Demux/3 -> Product2/1, Product1/1  "Az"
  b/1 -> Demux1/1
  a/1 -> Demux/1
  Add2/1 -> Vector Concatenate/3
  Demux/2 -> Product5/1, Product/1  "Ay"
  Demux1/3 -> Product/2, Product3/2  "Bz"
  Demux1/2 -> Product4/2, Product1/2  "By"
  Add1/1 -> Vector Concatenate/2

== system detumbling/Environment/Earth's Shadow/3D Norm ==
  V : Inport
  Add : Sum  Inputs=+++
  Demux : Demux  Outputs=3
  Square : Math  Operator=square  SaturateOnIntegerOverflow=on
  Square Root : Sqrt  SaturateOnIntegerOverflow=on
  Square1 : Math  Operator=square  SaturateOnIntegerOverflow=on
  Square2 : Math  Operator=square  SaturateOnIntegerOverflow=on
  normV : Outport
  wires:
  Square Root/1 -> normV/1
  V/1 -> Demux/1
  Demux/3 -> Square2/1
  Square/1 -> Add/1
  Demux/1 -> Square/1
  Demux/2 -> Square1/1
  Square2/1 -> Add/3
  Square1/1 -> Add/2
  Add/1 -> Square Root/1

== system detumbling/Environment/Gravity Gradient Torque/3D-Norm ==
  V : Inport
  Add : Sum  Inputs=+++
  Demux : Demux  Outputs=3
  Square : Math  Operator=square  SaturateOnIntegerOverflow=on
  Square Root : Sqrt  SaturateOnIntegerOverflow=on
  Square1 : Math  Operator=square  SaturateOnIntegerOverflow=on
  Square2 : Math  Operator=square  SaturateOnIntegerOverflow=on
  normV : Outport
  wires:
  Square Root/1 -> normV/1
  Add/1 -> Square Root/1
  Square2/1 -> Add/3
  Square1/1 -> Add/2
  Square/1 -> Add/1
  Demux/1 -> Square/1
  Demux/2 -> Square1/1
  Demux/3 -> Square2/1
  V/1 -> Demux/1

== system detumbling/Environment/Magnetic Torque/Cross Product ==
  a : Inport
  b : Inport  Port=2
  Add : Sum  Inputs=+-
  Add1 : Sum  Inputs=+-
  Add2 : Sum  Inputs=+-
  Demux : Demux  Outputs=3
  Demux1 : Demux  Outputs=3
  Product{,1..5} (6 alike) : Product
  Vector Concatenate : Concatenate  NumInputs=3
  c : Outport
  wires:
  Demux1/1 -> Product2/2, Product5/2  "Bx"
  Product2/1 -> Add1/1
  Vector Concatenate/1 -> c/1
  Add/1 -> Vector Concatenate/1
  Product3/1 -> Add1/2
  Product1/1 -> Add/2
  Product4/1 -> Add2/1
  Product/1 -> Add/1
  Demux/1 -> Product3/1, Product4/1  "Ax"
  Product5/1 -> Add2/2
  Demux/3 -> Product2/1, Product1/1  "Az"
  b/1 -> Demux1/1
  a/1 -> Demux/1
  Add2/1 -> Vector Concatenate/3
  Demux/2 -> Product5/1, Product/1  "Ay"
  Demux1/3 -> Product/2, Product3/2  "Bz"
  Demux1/2 -> Product4/2, Product1/2  "By"
  Add1/1 -> Vector Concatenate/2

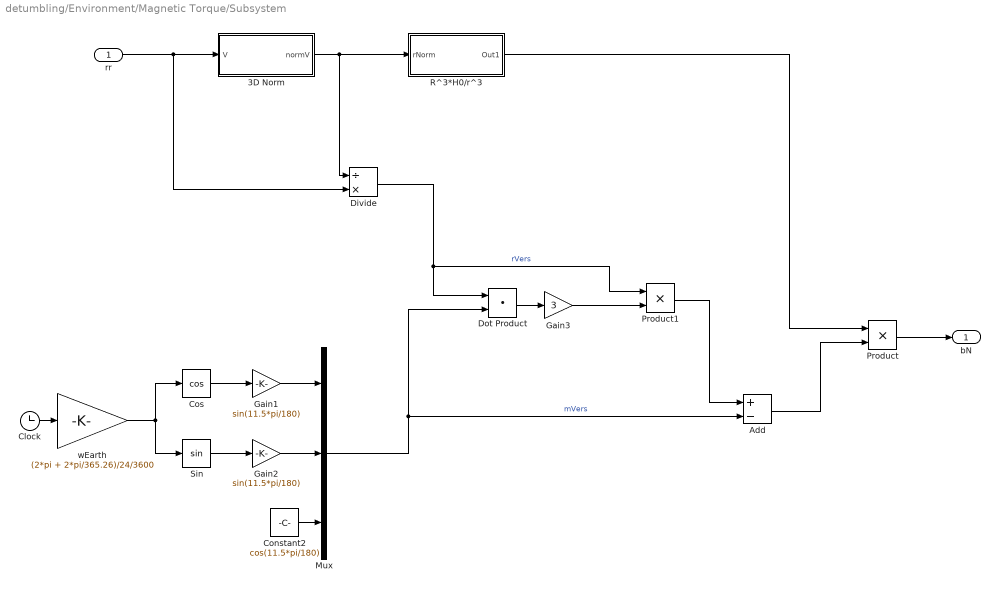
== system detumbling/Environment/Magnetic Torque/Subsystem ==
  rr : Inport
  3D Norm : Subsystem
  Add : Sum  Inputs=+-
  Clock : Clock
  Constant2 : Constant  Value=cos(11.5*pi/180)
  Cos : Trigonometry  Operator=cos
  Divide : Product  Inputs=/*
  Dot Product : DotProduct  InputSameDT=on  OutDataTypeStr=Inherit: Inherit via internal rule
  Gain1 : Gain  Gain=sin(11.5*pi/180)
  Gain2 : Gain  Gain=sin(11.5*pi/180)
  Gain3 : Gain  Gain=3
  Mux : Mux  Inputs=3
  Product : Product
  Product1 : Product
  R^3*H0/r^3 : Subsystem
  Sin : Trigonometry
  wEarth : Gain  Gain=(2*pi + 2*pi/365.26)/24/3600
  bN : Outport
  wires:
  3D Norm/1(normV) -> Divide/1, R^3*H0/r^3/1(rNorm)
  Cos/1 -> Gain1/1
  Sin/1 -> Gain2/1
  Gain2/1 -> Mux/2
  rr/1 -> 3D Norm/1(V), Divide/2
  Product1/1 -> Add/1
  wEarth/1 -> Sin/1, Cos/1
  Constant2/1 -> Mux/3
  Gain1/1 -> Mux/1
  Gain3/1 -> Product1/2
  Product/1 -> bN/1
  Add/1 -> Product/2
  Clock/1 -> wEarth/1
  R^3*H0/r^3/1(Out1) -> Product/1
  Dot Product/1 -> Gain3/1
  Divide/1 -> Product1/1, Dot Product/1  "rVers"
  Mux/1 -> Dot Product/2, Add/2  "mVers"

== system detumbling/Environment/Unperturbed Orbit/Subsystem ==
  theta : Inport
  Add : Sum
  Constant : Constant
  Cos : Trigonometry  Operator=cos
  Gain : Gain  Gain=data.orbit.e
  Gain1 : Gain  Gain=data.orbit.n/(1-data.orbit.e^2)^(3/2)
  Square : Math  Operator=square  SaturateOnIntegerOverflow=on
  theta_dot : Outport
  wires:
  theta/1 -> Cos/1
  Cos/1 -> Gain/1
  Gain/1 -> Add/1
  Constant/1 -> Add/2
  Add/1 -> Square/1
  Square/1 -> Gain1/1
  Gain1/1 -> theta_dot/1

== system detumbling/Environment/Unperturbed Orbit/Subsystem1 ==
  theta : Inport
  Build 3x3 Matrix : Subsystem
  Constant : Constant  Value=0
  Constant1 : Constant
  Cos1 : Trigonometry  Operator=cos
  Cos2 : Trigonometry  Operator=cos
  Gain : Gain  Gain=-1
  Gain1 : Gain  Gain=[1 0 0; 0 cos(data.orbit.i) sin(data.orbit.i); 0 -sin(data.orbit.i) cos(data.orbit.i)]  Multiplication=Matrix(u*K)
  Sin : Trigonometry
  Sin1 : Trigonometry
  ALN : Outport
  wires:
  Cos1/1 -> Build 3x3 Matrix/1(A11)
  theta/1 -> Cos2/1, Sin1/1, Cos1/1, Sin/1
  Sin/1 -> Gain/1
  Gain/1 -> Build 3x3 Matrix/2(A21)
  Sin1/1 -> Build 3x3 Matrix/4(A12)
  Cos2/1 -> Build 3x3 Matrix/5(A22)
  Constant/1 -> Build 3x3 Matrix/8(A23), Build 3x3 Matrix/7("A13 "), Build 3x3 Matrix/6(A32), Build 3x3 Matrix/3(A31)
  Constant1/1 -> Build 3x3 Matrix/9(A33)
  Build 3x3 Matrix/1(A) -> Gain1/1
  Gain1/1 -> ALN/1

== system detumbling/Environment/Unperturbed Orbit/Subsystem2 ==
  theta : Inport
  Add : Sum
  Constant : Constant
  Constant1 : Constant  Value=data.orbit.a*(1-data.orbit.e^2)
  Cos : Trigonometry  Operator=cos
  Cos1 : Trigonometry  Operator=cos
  Divide : Product  Inputs=/*
  Gain : Gain  Gain=cos(data.orbit.i)
  Gain1 : Gain  Gain=sin(data.orbit.i)
  Gain3 : Gain  Gain=data.orbit.e
  Mux : Mux  Inputs=3
  Product : Product
  Sin : Trigonometry
  Sin1 : Trigonometry
  rr : Outport
  wires:
  Cos/1 -> Mux/1
  theta/1 -> Cos1/1, Sin1/1, Cos/1, Sin/1
  Gain/1 -> Mux/2
  Gain1/1 -> Mux/3
  Sin/1 -> Gain/1
  Sin1/1 -> Gain1/1
  Cos1/1 -> Gain3/1
  Gain3/1 -> Add/1
  Constant/1 -> Add/2
  Add/1 -> Divide/1
  Constant1/1 -> Divide/2
  Divide/1 -> Product/2
  Mux/1 -> Product/1
  Product/1 -> rr/1

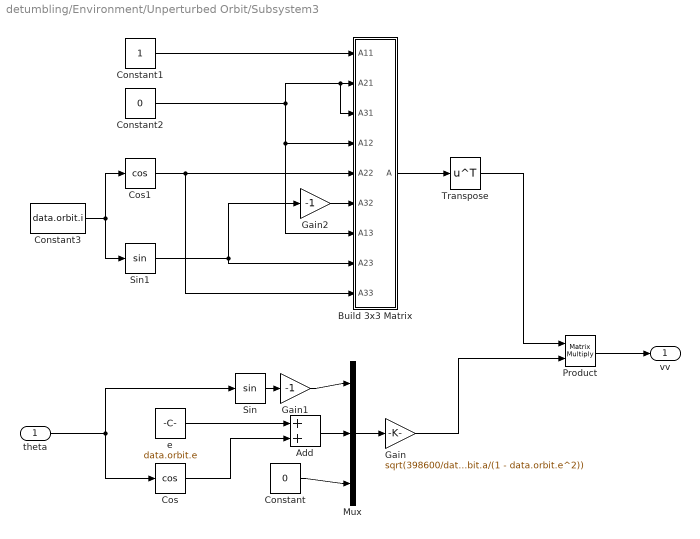
== system detumbling/Environment/Unperturbed Orbit/Subsystem3 ==
  theta : Inport
  Add : Sum
  Build 3x3 Matrix : Subsystem
  Constant : Constant  Value=0
  Constant1 : Constant
  Constant2 : Constant  Value=0
  Constant3 : Constant  Value=data.orbit.i
  Cos : Trigonometry  Operator=cos
  Cos1 : Trigonometry  Operator=cos
  Gain : Gain  Gain=sqrt(398600/data.orbit.a/(1 - data.orbit.e^2))
  Gain1 : Gain  Gain=-1
  Gain2 : Gain  Gain=-1
  Mux : Mux  Inputs=3
  Product : Product  Multiplication=Matrix(*)
  Sin : Trigonometry
  Sin1 : Trigonometry
  Transpose : Math  Operator=transpose  SaturateOnIntegerOverflow=on
  e : Constant  Value=data.orbit.e
  vv : Outport
  wires:
  Mux/1 -> Gain/1
  theta/1 -> Cos/1, Sin/1
  Constant/1 -> Mux/3
  Add/1 -> Mux/2
  Cos/1 -> Add/2
  Sin/1 -> Gain1/1
  e/1 -> Add/1
  Gain1/1 -> Mux/1
  Constant3/1 -> Sin1/1, Cos1/1
  Constant1/1 -> Build 3x3 Matrix/1(A11)
  Constant2/1 -> Build 3x3 Matrix/3(A31), Build 3x3 Matrix/2(A21), Build 3x3 Matrix/4(A12), Build 3x3 Matrix/7("A13 ")
  Cos1/1 -> Build 3x3 Matrix/9(A33), Build 3x3 Matrix/5(A22)
  Gain2/1 -> Build 3x3 Matrix/6(A32)
  Sin1/1 -> Build 3x3 Matrix/8(A23), Gain2/1
  Build 3x3 Matrix/1(A) -> Transpose/1
  Transpose/1 -> Product/1
  Gain/1 -> Product/2
  Product/1 -> vv/1

== system detumbling/Nonlinear Observer/Observer/Cross Product ==
  a : Inport
  b : Inport  Port=2
  Add : Sum  Inputs=+-
  Add1 : Sum  Inputs=+-
  Add2 : Sum  Inputs=+-
  Demux : Demux  Outputs=3
  Demux1 : Demux  Outputs=3
  Product{,1..5} (6 alike) : Product
  Vector Concatenate : Concatenate  NumInputs=3
  c : Outport
  wires:
  Demux1/1 -> Product2/2, Product5/2  "Bx"
  Product2/1 -> Add1/1
  Vector Concatenate/1 -> c/1
  Add/1 -> Vector Concatenate/1
  Product3/1 -> Add1/2
  Product1/1 -> Add/2
  Product4/1 -> Add2/1
  Product/1 -> Add/1
  Demux/1 -> Product3/1, Product4/1  "Ax"
  Product5/1 -> Add2/2
  Demux/3 -> Product2/1, Product1/1  "Az"
  b/1 -> Demux1/1
  a/1 -> Demux/1
  Add2/1 -> Vector Concatenate/3
  Demux/2 -> Product5/1, Product/1  "Ay"
  Demux1/3 -> Product/2, Product3/2  "Bz"
  Demux1/2 -> Product4/2, Product1/2  "By"
  Add1/1 -> Vector Concatenate/2

== system detumbling/Environment/Magnetic Torque/Subsystem/3D Norm ==
  V : Inport
  Add : Sum  Inputs=+++
  Demux : Demux  Outputs=3
  Square : Math  Operator=square  SaturateOnIntegerOverflow=on
  Square Root : Sqrt  SaturateOnIntegerOverflow=on
  Square1 : Math  Operator=square  SaturateOnIntegerOverflow=on
  Square2 : Math  Operator=square  SaturateOnIntegerOverflow=on
  normV : Outport
  wires:
  Square Root/1 -> normV/1
  V/1 -> Demux/1
  Demux/3 -> Square2/1
  Square/1 -> Add/1
  Demux/1 -> Square/1
  Demux/2 -> Square1/1
  Square2/1 -> Add/3
  Square1/1 -> Add/2
  Add/1 -> Square Root/1

== system detumbling/Environment/Magnetic Torque/Subsystem/R^3*H0//r^3 ==
  rNorm : Inport
  Constant : Constant  Value=3
  Constant1 : Constant  Value=3
  Divide : Product  Inputs=**/
  H0 : Constant  Value=((-29615e-9)^2 + (-1728e-9)^2 + 5186e-9^2)^(1/2)
  Power : Math  Operator=pow  SaturateOnIntegerOverflow=on
  Power1 : Math  Operator=pow  SaturateOnIntegerOverflow=on
  R_EARTH : Constant  Value=6371
  Out1 : Outport
  wires:
  H0/1 -> Divide/2
  Power/1 -> Divide/1
  Power1/1 -> Divide/3
  Divide/1 -> Out1/1
  Constant1/1 -> Power1/2
  rNorm/1 -> Power1/1
  Constant/1 -> Power/2
  R_EARTH/1 -> Power/1

== system detumbling/Environment/Unperturbed Orbit/Subsystem1/Build 3x3 Matrix ==
  A11 : Inport
  A21 : Inport  Port=2
  A31 : Inport  Port=3
  A12 : Inport  Port=4
  A22 : Inport  Port=5
  A32 : Inport  Port=6
  "A13 " : Inport  Port=7
  A23 : Inport  Port=8
  A33 : Inport  Port=9
  Mux : Mux  Inputs=3
  Mux1 : Mux  Inputs=3
  Mux2 : Mux  Inputs=3
  Vector Concatenate : Concatenate  NumInputs=3  Mode=Multidimensional array  ConcatenateDimension=2
  A : Outport
  wires:
  A21/1 -> Mux/2
  A23/1 -> Mux2/2
  "A13 "/1 -> Mux2/1
  A11/1 -> Mux/1
  Vector Concatenate/1 -> A/1
  A31/1 -> Mux/3
  A12/1 -> Mux1/1
  A22/1 -> Mux1/2
  Mux2/1 -> Vector Concatenate/3
  Mux1/1 -> Vector Concatenate/2
  Mux/1 -> Vector Concatenate/1
  A33/1 -> Mux2/3
  A32/1 -> Mux1/3

== system detumbling/Environment/Unperturbed Orbit/Subsystem3/Build 3x3 Matrix ==
  A11 : Inport
  A21 : Inport  Port=2
  A31 : Inport  Port=3
  A12 : Inport  Port=4
  A22 : Inport  Port=5
  A32 : Inport  Port=6
  "A13 " : Inport  Port=7
  A23 : Inport  Port=8
  A33 : Inport  Port=9
  Mux : Mux  Inputs=3
  Mux1 : Mux  Inputs=3
  Mux2 : Mux  Inputs=3
  Vector Concatenate : Concatenate  NumInputs=3  Mode=Multidimensional array  ConcatenateDimension=2
  A : Outport
  wires:
  A21/1 -> Mux/2
  A23/1 -> Mux2/2
  "A13 "/1 -> Mux2/1
  A11/1 -> Mux/1
  Vector Concatenate/1 -> A/1
  A31/1 -> Mux/3
  A12/1 -> Mux1/1
  A22/1 -> Mux1/2
  Mux2/1 -> Vector Concatenate/3
  Mux1/1 -> Vector Concatenate/2
  Mux/1 -> Vector Concatenate/1
  A33/1 -> Mux2/3
  A32/1 -> Mux1/3

== matlab function detumbling/Environment/Drag ==
  data: NBMat input; M output; rSurf input; aSurf input; cd input; rho input; rr input; vv input; ABN input
function M = fcn(NBMat,rSurf,aSurf,cd,rho,rr,vv,ABN)

wEarth = 0.000072921;

rr = rr*1e3; vv = vv*1e3;

vRel = ABN*[vv(1) + wEarth*rr(1); vv(2) - wEarth*rr(2); vv(3)];

nSurf = size(NBMat,2);

M = [0; 0; 0];

for i = 1:nSurf
    
    NBi = NBMat(:,i); ri = rSurf(:,i); Ai = aSurf(i);
    
    Ki = dot(vRel/norm(vRel),NBi); 
    
    if Ki > 0
        
        Fi = -0.5*rho*cd*norm(vRel)*vRel*Ai*Ki;
        
        M = M + cross(ri,Fi);
        
    end
    
end

end

== matlab function detumbling/Environment/MATLAB Function ==
  data: SB input; isInEarthShadow input; rhoS input; rhoD input; NBMat input; rSurf input; aSurf input; M output
function M = SRP(SB,isInEarthShadow,rhoS,rhoD,NBMat,rSurf,aSurf)

% Constants:
Fe = 1975; c = 3e8; P = Fe/c;

nSurf = size(NBMat,2);

M = [0; 0; 0];

if ~isInEarthShadow
    
    for i = 1:nSurf
        
        NBi = NBMat(:,i); ri = rSurf(:,i); Ai = aSurf(i);
        rhoSi = rhoS(i); rhoDi = rhoD(i);
        
        Ki = dot(SB,NBi);
        
        if Ki > 0
            
            Fi = -P*Ai*Ki*((1-rhoSi)*SB +...
                (2*rhoSi*Ki + 2/3*rhoDi)*NBi);
            
            M = M + cross(ri,Fi);
            
        end
        
    end
    
end
end
